simulink model "PubIfDecisionTOS_MDL"  (R2020b)
settings: configuration reference "DspaceConfig" (kept outside this file)
PostLoadFcn:
  | if any(exist('dsrtsu_mdlpostloadfcn', 'file') ~= 0), dsrtsu_mdlpostloadfcn('Execute', bdroot); end
InitFcn:
  | , if any(exist('dsmpb_private', 'file') ~= 0), dsmpb_private('dsmpb_mdlclblib', 'Init', bdroot); end,
undefined symbols (not defined in the file or in its folder): C_TOS_ACCEgoRAxletoFbumplength_m, C_TOS_ACCTargetFront_Flag, C_TOS_AEBJAPedObjDxThre_Val, C_TOS_AEBJAPedObjDyThre_Val, C_TOS_AEBJATargetSize_Val, C_TOS_AEBJAVehObjDxThre_Val, C_TOS_AEBJAVehObjDyThre_Val, C_TOS_AEBJuncPedTargetSize_Val, C_TOS_AEBLatObjDxThre_Val, C_TOS_AEBLatPedDyThre_Val, C_TOS_AEBLatTargetSize_Val, C_TOS_AEBLongTargetInEgoFront_Flag, C_TOS_axAbsGround_Parameter, C_TOS_CameraConfirmedFlag, C_TOS_CNsubjWidth, C_TOS_CurrentLaneCoreMinWidth_Val, C_TOS_CutInProb_Val_Zero, C_TOS_CutOutProb_Val_Zero, C_TOS_D2R_Val, C_TOS_DefaultValueObjectToCenterLine_dy, C_TOS_EgoCarWidth_Val, C_TOS_EgoDxRefPoint_m, C_TOS_EgoRAxletoFbumplength_m, C_TOS_HalfWidthVehicle_Con, C_TOS_HWA_CurrentLaneFlag, C_TOS_HWA_LeftLaneFlag, C_TOS_HWA_MovingDir_Vaild, C_TOS_HWA_MovState_Vaild, C_TOS_HWA_RightLaneFlag, C_TOS_LaneLineCourseErrorFront, C_TOS_LaneLineCourseErrorRear, C_TOS_MotorbikeDefaultWidth_m, C_TOS_NumberOfEffectiveTargets, C_TOS_Obj_Age_Val, C_TOS_Objdx_Constraint_Val, C_TOS_ObjectDefaultWidth_m, C_TOS_ObjInCurrentLane_Val, C_TOS_ObjInCurrentLaneValid, C_TOS_ObjInLeftLaneValid, C_TOS_ObjInRightLaneValid, C_TOS_ObjNotInCurrentLane_Val, C_TOS_ObjNotREElementType, C_TOS_ObjPredictDis_dy_ConstantVal_Zeros, C_TOS_ObjToCenterLine_ConstantVal_Zeros, C_TOS_OFMObjIDInvilad_Val, C_TOS_PIL_LatDisCons_Val_zero, C_TOS_PIL_ObjectCutInFlag_b, C_TOS_PIL_ObjectCutOutFlag_b, C_TOS_PIL_ObjLaneProb_al_Val, C_TOS_PP_ObjFusType_FC_Confirm_b, C_TOS_PP_ObjFusType_FC_FR_Confirm_b, C_TOS_PP_ObjFusType_FR_Confirm_b, C_TOS_RE_80BoolDefault_Val, C_TOS_RE_80Single181Default_Val, C_TOS_RE_80Single255Default_Val, C_TOS_RE_80Uint8Default_Val, C_TOS_RE_D2R, C_TOS_RE_D_180_Val, C_TOS_RE_InvalidObjectID_Val, C_TOS_RE_InvalidTargetChainDir_Val ... (+142)
libraries: simulink x1650, TOS_LIB x361, canfdmsglib x14
(part 61 of 69)

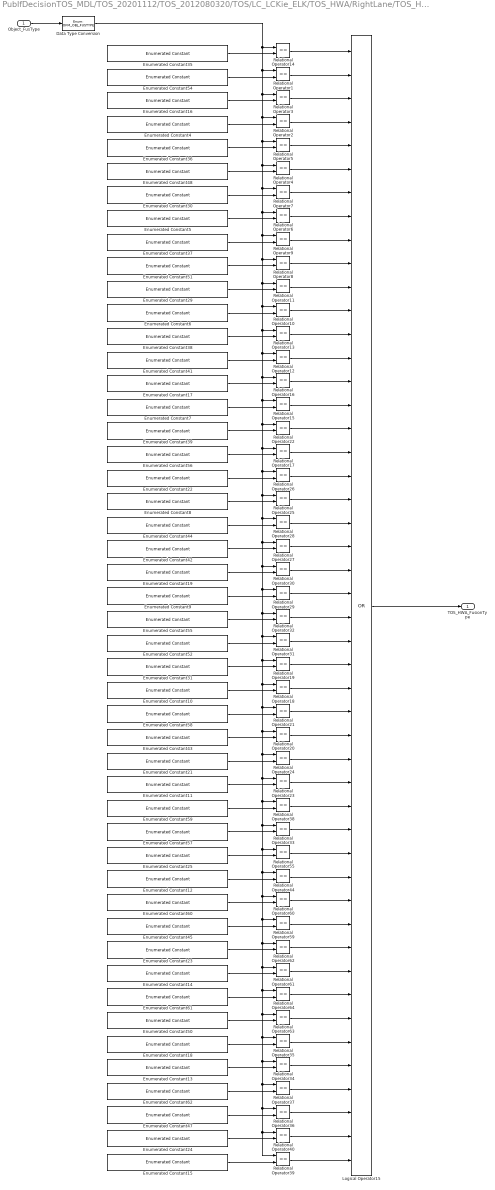
== system PubIfDecisionTOS_MDL/TOS_20201112/TOS_2012080320/TOS/LC_LCKie_ELK/TOS_HWA/RightLane/TOS_HWA_RightLane/TOS_HWA_RightLane/TOS_HWA/HWA_RightLane/HWA_RightLane_Rear/HWA_RightRear_FusionType/FusionType ==
  Object_FusType : Inport
  Data Type Conversion : DataTypeConversion  OutDataTypeStr=Enum: OFM_OBJ_FUSTYPE
  Enumerated Constant10 : simulink/Sources/Enumerated Constant  OutDataTypeStr=Enum: OFM_OBJ_FUSTYPE  Value=OFM_OBJ_FUSTYPE.FC_FR_CR_BR  SampleTime=inf
      settings: AttributesFormatString=OFM_OBJ_FUSTYPE.FC_FR_CR_BR=43
  Enumerated Constant11 : simulink/Sources/Enumerated Constant  OutDataTypeStr=Enum: OFM_OBJ_FUSTYPE  Value=OFM_OBJ_FUSTYPE.FC_FR_CL_CR_BR  SampleTime=inf
      settings: AttributesFormatString=OFM_OBJ_FUSTYPE.FC_FR_CL_CR_BR=47
  Enumerated Constant12 : simulink/Sources/Enumerated Constant  OutDataTypeStr=Enum: OFM_OBJ_FUSTYPE  Value=OFM_OBJ_FUSTYPE.FC_FR_BL_BR  SampleTime=inf
      settings: AttributesFormatString=OFM_OBJ_FUSTYPE.FC_FR_BL_BR=51
  Enumerated Constant13 : simulink/Sources/Enumerated Constant  OutDataTypeStr=Enum: OFM_OBJ_FUSTYPE  Value=OFM_OBJ_FUSTYPE.FC_FR_CR_BL_BR  SampleTime=inf
      settings: AttributesFormatString=OFM_OBJ_FUSTYPE.FC_FR_CR_BL_BR=59
  Enumerated Constant14 : simulink/Sources/Enumerated Constant  OutDataTypeStr=Enum: OFM_OBJ_FUSTYPE  Value=OFM_OBJ_FUSTYPE.FC_FR_CL_BL_BR  SampleTime=inf
      settings: AttributesFormatString=OFM_OBJ_FUSTYPE.FC_FR_CL_BL_BR=55
  Enumerated Constant15 : simulink/Sources/Enumerated Constant  OutDataTypeStr=Enum: OFM_OBJ_FUSTYPE  Value=OFM_OBJ_FUSTYPE.FC_FR_CL_CR_BL_BR  SampleTime=inf
      settings: AttributesFormatString=OFM_OBJ_FUSTYPE.FC_FR_CL_CR_BL_BR=63
  Enumerated Constant16 : simulink/Sources/Enumerated Constant  OutDataTypeStr=Enum: OFM_OBJ_FUSTYPE  Value=OFM_OBJ_FUSTYPE.FR_BL  SampleTime=inf
      settings: AttributesFormatString=OFM_OBJ_FUSTYPE.FR_BL = 18
  Enumerated Constant17 : simulink/Sources/Enumerated Constant  OutDataTypeStr=Enum: OFM_OBJ_FUSTYPE  Value=OFM_OBJ_FUSTYPE.FR_CL_CR_BL  SampleTime=inf
      settings: AttributesFormatString=OFM_OBJ_FUSTYPE.FR_CL_CR_BL = 30
  Enumerated Constant18 : simulink/Sources/Enumerated Constant  OutDataTypeStr=Enum: OFM_OBJ_FUSTYPE  Value=OFM_OBJ_FUSTYPE.FR_CR_BL_BR  SampleTime=inf
      settings: AttributesFormatString=OFM_OBJ_FUSTYPE.FR_CR_BL_BR = 58
  Enumerated Constant19 : simulink/Sources/Enumerated Constant  OutDataTypeStr=Enum: OFM_OBJ_FUSTYPE  Value=OFM_OBJ_FUSTYPE.FR_CL_BR  SampleTime=inf
      settings: AttributesFormatString=OFM_OBJ_FUSTYPE.FR_CL_BR = 38
  Enumerated Constant21 : simulink/Sources/Enumerated Constant  OutDataTypeStr=Enum: OFM_OBJ_FUSTYPE  Value=OFM_OBJ_FUSTYPE.FR_CL_CR_BR  SampleTime=inf
      settings: AttributesFormatString=OFM_OBJ_FUSTYPE.FR_CL_CR_BR = 46
  Enumerated Constant22 : simulink/Sources/Enumerated Constant  OutDataTypeStr=Enum: OFM_OBJ_FUSTYPE  Value=OFM_OBJ_FUSTYPE.FR_BR  SampleTime=inf
      settings: AttributesFormatString=OFM_OBJ_FUSTYPE.FR_BR = 34
  Enumerated Constant23 : simulink/Sources/Enumerated Constant  OutDataTypeStr=Enum: OFM_OBJ_FUSTYPE  Value=OFM_OBJ_FUSTYPE.FR_CL_BL_BR  SampleTime=inf
      settings: AttributesFormatString=OFM_OBJ_FUSTYPE.FR_CL_BL_BR = 54
  Enumerated Constant24 : simulink/Sources/Enumerated Constant  OutDataTypeStr=Enum: OFM_OBJ_FUSTYPE  Value=OFM_OBJ_FUSTYPE.FR_CL_CR_BL_BR  SampleTime=inf
      settings: AttributesFormatString=OFM_OBJ_FUSTYPE.FR_CL_CR_BL_BR = 62
  Enumerated Constant25 : simulink/Sources/Enumerated Constant  OutDataTypeStr=Enum: OFM_OBJ_FUSTYPE  Value=OFM_OBJ_FUSTYPE.FR_BL_BR  SampleTime=inf
      settings: AttributesFormatString=OFM_OBJ_FUSTYPE.FR_BL_BR = 50
  Enumerated Constant29 : simulink/Sources/Enumerated Constant  OutDataTypeStr=Enum: OFM_OBJ_FUSTYPE  Value=OFM_OBJ_FUSTYPE.FR_CR_BL  SampleTime=inf
      settings: AttributesFormatString=OFM_OBJ_FUSTYPE.FR_CR_BL = 26
  Enumerated Constant30 : simulink/Sources/Enumerated Constant  OutDataTypeStr=Enum: OFM_OBJ_FUSTYPE  Value=OFM_OBJ_FUSTYPE.FR_CL_BL  SampleTime=inf
      settings: AttributesFormatString=OFM_OBJ_FUSTYPE.FR_CL_BL = 22
  Enumerated Constant31 : simulink/Sources/Enumerated Constant  OutDataTypeStr=Enum: OFM_OBJ_FUSTYPE  Value=OFM_OBJ_FUSTYPE.FR_CR_BR  SampleTime=inf
      settings: AttributesFormatString=OFM_OBJ_FUSTYPE.FR_CR_BR = 42
  Enumerated Constant35 : simulink/Sources/Enumerated Constant  OutDataTypeStr=Enum: OFM_OBJ_FUSTYPE  Value=OFM_OBJ_FUSTYPE.BL  SampleTime=inf
      settings: AttributesFormatString=OFM_OBJ_FUSTYPE.BL = 16
  Enumerated Constant36 : simulink/Sources/Enumerated Constant  OutDataTypeStr=Enum: OFM_OBJ_FUSTYPE  Value=OFM_OBJ_FUSTYPE.CL_BL  SampleTime=inf
      settings: AttributesFormatString=OFM_OBJ_FUSTYPE.CL_BL=20
  Enumerated Constant37 : simulink/Sources/Enumerated Constant  OutDataTypeStr=Enum: OFM_OBJ_FUSTYPE  Value=OFM_OBJ_FUSTYPE.CR_BL  SampleTime=inf
      settings: AttributesFormatString=OFM_OBJ_FUSTYPE.CR_BL = 24
  Enumerated Constant38 : simulink/Sources/Enumerated Constant  OutDataTypeStr=Enum: OFM_OBJ_FUSTYPE  Value=OFM_OBJ_FUSTYPE.CL_CR_BL  SampleTime=inf
      settings: AttributesFormatString=OFM_OBJ_FUSTYPE.CL_CR_BL=28
  Enumerated Constant39 : simulink/Sources/Enumerated Constant  OutDataTypeStr=Enum: OFM_OBJ_FUSTYPE  Value=OFM_OBJ_FUSTYPE.BR  SampleTime=inf
      settings: AttributesFormatString=OFM_OBJ_FUSTYPE.BR = 32
  Enumerated Constant4 : simulink/Sources/Enumerated Constant  OutDataTypeStr=Enum: OFM_OBJ_FUSTYPE  Value=OFM_OBJ_FUSTYPE.FC_FR_BL  SampleTime=inf
      settings: AttributesFormatString=OFM_OBJ_FUSTYPE.FC_FR_BL=19
  Enumerated Constant41 : simulink/Sources/Enumerated Constant  OutDataTypeStr=Enum: OFM_OBJ_FUSTYPE  Value=OFM_OBJ_FUSTYPE.FC_CL_CR_BL  SampleTime=inf
      settings: AttributesFormatString=OFM_OBJ_FUSTYPE.FC_CL_CR_BL = 29
  Enumerated Constant42 : simulink/Sources/Enumerated Constant  OutDataTypeStr=Enum: OFM_OBJ_FUSTYPE  Value=OFM_OBJ_FUSTYPE.FC_CL_BR  SampleTime=inf
      settings: AttributesFormatString=OFM_OBJ_FUSTYPE.FC_CL_BR = 37
  Enumerated Constant43 : simulink/Sources/Enumerated Constant  OutDataTypeStr=Enum: OFM_OBJ_FUSTYPE  Value=OFM_OBJ_FUSTYPE.FC_CL_CR_BR  SampleTime=inf
      settings: AttributesFormatString=OFM_OBJ_FUSTYPE.FC_CL_CR_BR = 45
  Enumerated Constant44 : simulink/Sources/Enumerated Constant  OutDataTypeStr=Enum: OFM_OBJ_FUSTYPE  Value=OFM_OBJ_FUSTYPE.CL_BR  SampleTime=inf
      settings: AttributesFormatString=OFM_OBJ_FUSTYPE.CL_BR = 36
  Enumerated Constant45 : simulink/Sources/Enumerated Constant  OutDataTypeStr=Enum: OFM_OBJ_FUSTYPE  Value=OFM_OBJ_FUSTYPE.FC_CL_BL_BR  SampleTime=inf
      settings: AttributesFormatString=OFM_OBJ_FUSTYPE.FC_CL_BL_BR = 53
  Enumerated Constant47 : simulink/Sources/Enumerated Constant  OutDataTypeStr=Enum: OFM_OBJ_FUSTYPE  Value=OFM_OBJ_FUSTYPE.FC_CL_CR_BL_BR  SampleTime=inf
      settings: AttributesFormatString=OFM_OBJ_FUSTYPE.FC_CL_CR_BL_BR = 61
  Enumerated Constant48 : simulink/Sources/Enumerated Constant  OutDataTypeStr=Enum: OFM_OBJ_FUSTYPE  Value=OFM_OBJ_FUSTYPE.FC_CL_BL  SampleTime=inf
      settings: AttributesFormatString=OFM_OBJ_FUSTYPE.FC_CL_BL = 21
  Enumerated Constant5 : simulink/Sources/Enumerated Constant  OutDataTypeStr=Enum: OFM_OBJ_FUSTYPE  Value=OFM_OBJ_FUSTYPE.FC_FR_CL_BL  SampleTime=inf
      settings: AttributesFormatString=OFM_OBJ_FUSTYPE.FC_FR_CL_BL=23
  Enumerated Constant50 : simulink/Sources/Enumerated Constant  OutDataTypeStr=Enum: OFM_OBJ_FUSTYPE  Value=OFM_OBJ_FUSTYPE.FC_CR_BL_BR  SampleTime=inf
      settings: AttributesFormatString=OFM_OBJ_FUSTYPE.FC_CR_BL_BR = 57
  Enumerated Constant51 : simulink/Sources/Enumerated Constant  OutDataTypeStr=Enum: OFM_OBJ_FUSTYPE  Value=OFM_OBJ_FUSTYPE.FC_CR_BL  SampleTime=inf
      settings: AttributesFormatString=OFM_OBJ_FUSTYPE.FC_CR_BL = 25
  Enumerated Constant52 : simulink/Sources/Enumerated Constant  OutDataTypeStr=Enum: OFM_OBJ_FUSTYPE  Value=OFM_OBJ_FUSTYPE.FC_CR_BR  SampleTime=inf
      settings: AttributesFormatString=OFM_OBJ_FUSTYPE.FC_CR_BR = 41
  Enumerated Constant54 : simulink/Sources/Enumerated Constant  OutDataTypeStr=Enum: OFM_OBJ_FUSTYPE  Value=OFM_OBJ_FUSTYPE.FC_BL  SampleTime=inf
      settings: AttributesFormatString=OFM_OBJ_FUSTYPE.FC_BL = 17
  Enumerated Constant55 : simulink/Sources/Enumerated Constant  OutDataTypeStr=Enum: OFM_OBJ_FUSTYPE  Value=OFM_OBJ_FUSTYPE.CR_BR  SampleTime=inf
      settings: AttributesFormatString=OFM_OBJ_FUSTYPE.CR_BR = 40
  Enumerated Constant56 : simulink/Sources/Enumerated Constant  OutDataTypeStr=Enum: OFM_OBJ_FUSTYPE  Value=OFM_OBJ_FUSTYPE.FC_BR  SampleTime=inf
      settings: AttributesFormatString=OFM_OBJ_FUSTYPE.FC_BR = 33
  Enumerated Constant57 : simulink/Sources/Enumerated Constant  OutDataTypeStr=Enum: OFM_OBJ_FUSTYPE  Value=OFM_OBJ_FUSTYPE.FC_BL_BR  SampleTime=inf
      settings: AttributesFormatString=OFM_OBJ_FUSTYPE.FC_BL_BR = 49
  Enumerated Constant58 : simulink/Sources/Enumerated Constant  OutDataTypeStr=Enum: OFM_OBJ_FUSTYPE  Value=OFM_OBJ_FUSTYPE.CL_CR_BR  SampleTime=inf
      settings: AttributesFormatString=OFM_OBJ_FUSTYPE.CL_CR_BR = 44
  Enumerated Constant59 : simulink/Sources/Enumerated Constant  OutDataTypeStr=Enum: OFM_OBJ_FUSTYPE  Value=OFM_OBJ_FUSTYPE.BL_BR  SampleTime=inf
      settings: AttributesFormatString=OFM_OBJ_FUSTYPE.BL_BR = 48
  Enumerated Constant6 : simulink/Sources/Enumerated Constant  OutDataTypeStr=Enum: OFM_OBJ_FUSTYPE  Value=OFM_OBJ_FUSTYPE.FC_FR_CR_BL  SampleTime=inf
      settings: AttributesFormatString=OFM_OBJ_FUSTYPE.FC_FR_CR_BL=27
  Enumerated Constant60 : simulink/Sources/Enumerated Constant  OutDataTypeStr=Enum: OFM_OBJ_FUSTYPE  Value=OFM_OBJ_FUSTYPE.CL_BL_BR  SampleTime=inf
      settings: AttributesFormatString=OFM_OBJ_FUSTYPE.CL_BL_BR = 52
  Enumerated Constant61 : simulink/Sources/Enumerated Constant  OutDataTypeStr=Enum: OFM_OBJ_FUSTYPE  Value=OFM_OBJ_FUSTYPE.CR_BL_BR  SampleTime=inf
      settings: AttributesFormatString=OFM_OBJ_FUSTYPE.CR_BL_BR = 56
  Enumerated Constant62 : simulink/Sources/Enumerated Constant  OutDataTypeStr=Enum: OFM_OBJ_FUSTYPE  Value=OFM_OBJ_FUSTYPE.CL_CR_BL_BR  SampleTime=inf
      settings: AttributesFormatString=OFM_OBJ_FUSTYPE.CL_CR_BL_BR = 60
  Enumerated Constant7 : simulink/Sources/Enumerated Constant  OutDataTypeStr=Enum: OFM_OBJ_FUSTYPE  Value=OFM_OBJ_FUSTYPE.FC_FR_CL_CR_BL  SampleTime=inf
      settings: AttributesFormatString=OFM_OBJ_FUSTYPE.FC_FR_CL_CR_BL=31
  Enumerated Constant8 : simulink/Sources/Enumerated Constant  OutDataTypeStr=Enum: OFM_OBJ_FUSTYPE  Value=OFM_OBJ_FUSTYPE.FC_FR_BR  SampleTime=inf
      settings: AttributesFormatString=OFM_OBJ_FUSTYPE.FC_FR_BR=35
  Enumerated Constant9 : simulink/Sources/Enumerated Constant  OutDataTypeStr=Enum: OFM_OBJ_FUSTYPE  Value=OFM_OBJ_FUSTYPE.FC_FR_CL_BR  SampleTime=inf
      settings: AttributesFormatString=OFM_OBJ_FUSTYPE.FC_FR_CL_BR=39
  Logical Operator15 : Logic  Operator=OR  Inputs=48  AllPortsSameDT=off  OutDataTypeStr=boolean
  Relational Operator{1..40,44,55,59..64} (48 alike) : RelationalOperator  Operator===  OutDataTypeStr=boolean  RndMeth=Nearest
  TOS_HWA_FusionType : Outport
  wires:
  Relational Operator29/1 -> Logical Operator15/24
  Enumerated Constant50/1 -> Relational Operator63/2
  Enumerated Constant15/1 -> Relational Operator39/2
  Relational Operator8/1 -> Logical Operator15/10
  Relational Operator27/1 -> Logical Operator15/22
  Relational Operator7/1 -> Logical Operator15/7
  Enumerated Constant54/1 -> Relational Operator1/2
  Enumerated Constant58/1 -> Relational Operator21/2
  Relational Operator16/1 -> Logical Operator15/15
  Enumerated Constant44/1 -> Relational Operator28/2
  Enumerated Constant48/1 -> Relational Operator4/2
  Enumerated Constant23/1 -> Relational Operator62/2
  Relational Operator28/1 -> Logical Operator15/21
  Logical Operator15/1 -> TOS_HWA_FusionType/1
  Relational Operator23/1 -> Logical Operator15/32
  Relational Operator13/1 -> Logical Operator15/13
  Relational Operator3/1 -> Logical Operator15/3
  Relational Operator38/1 -> Logical Operator15/33
  Enumerated Constant16/1 -> Relational Operator3/2
  Enumerated Constant4/1 -> Relational Operator2/2
  Relational Operator9/1 -> Logical Operator15/9
  Enumerated Constant57/1 -> Relational Operator33/2
  Relational Operator33/1 -> Logical Operator15/34
  Enumerated Constant19/1 -> Relational Operator30/2
  Enumerated Constant30/1 -> Relational Operator7/2
  Relational Operator17/1 -> Logical Operator15/18
  Relational Operator25/1 -> Logical Operator15/20
  Relational Operator1/1 -> Logical Operator15/2
  Enumerated Constant41/1 -> Relational Operator12/2
  Enumerated Constant7/1 -> Relational Operator15/2
  Relational Operator64/1 -> Logical Operator15/41
  Relational Operator35/1 -> Logical Operator15/43
  Relational Operator63/1 -> Logical Operator15/42
  Enumerated Constant6/1 -> Relational Operator10/2
  Relational Operator44/1 -> Logical Operator15/36
  Relational Operator34/1 -> Logical Operator15/44
  Relational Operator15/1 -> Logical Operator15/16
  Relational Operator59/1 -> Logical Operator15/38
  Enumerated Constant22/1 -> Relational Operator26/2
  Relational Operator22/1 -> Logical Operator15/17
  Enumerated Constant35/1 -> Relational Operator14/2
  Enumerated Constant37/1 -> Relational Operator9/2
  Enumerated Constant59/1 -> Relational Operator38/2
  Enumerated Constant21/1 -> Relational Operator24/2
  Relational Operator6/1 -> Logical Operator15/8
  Enumerated Constant9/1 -> Relational Operator29/2
  Relational Operator11/1 -> Logical Operator15/11
  Relational Operator26/1 -> Logical Operator15/19
  Relational Operator60/1 -> Logical Operator15/37
  Enumerated Constant45/1 -> Relational Operator59/2
  Relational Operator18/1 -> Logical Operator15/28
  Enumerated Constant12/1 -> Relational Operator44/2
  Enumerated Constant11/1 -> Relational Operator23/2
  Enumerated Constant14/1 -> Relational Operator61/2
  Relational Operator36/1 -> Logical Operator15/46
  Relational Operator20/1 -> Logical Operator15/30
  Enumerated Constant31/1 -> Relational Operator19/2
  Enumerated Constant55/1 -> Relational Operator32/2
  Enumerated Constant43/1 -> Relational Operator20/2
  Relational Operator61/1 -> Logical Operator15/40
  Relational Operator19/1 -> Logical Operator15/27
  Enumerated Constant18/1 -> Relational Operator35/2
  Enumerated Constant5/1 -> Relational Operator6/2
  Relational Operator10/1 -> Logical Operator15/12
  Enumerated Constant25/1 -> Relational Operator55/2
  Relational Operator24/1 -> Logical Operator15/31
  Relational Operator21/1 -> Logical Operator15/29
  Enumerated Constant60/1 -> Relational Operator60/2
  Enumerated Constant61/1 -> Relational Operator64/2
  Relational Operator40/1 -> Logical Operator15/47
  Relational Operator2/1 -> Logical Operator15/4
  Relational Operator4/1 -> Logical Operator15/6
  Enumerated Constant8/1 -> Relational Operator25/2
  Enumerated Constant47/1 -> Relational Operator36/2
  Enumerated Constant13/1 -> Relational Operator34/2
  Enumerated Constant38/1 -> Relational Operator13/2
  Relational Operator37/1 -> Logical Operator15/45
  Object_FusType/1 -> Data Type Conversion/1
  Relational Operator5/1 -> Logical Operator15/5
  Relational Operator32/1 -> Logical Operator15/25
  Relational Operator39/1 -> Logical Operator15/48
  Enumerated Constant24/1 -> Relational Operator40/2
  Enumerated Constant51/1 -> Relational Operator8/2
  Enumerated Constant29/1 -> Relational Operator11/2
  Enumerated Constant56/1 -> Relational Operator17/2
  Enumerated Constant52/1 -> Relational Operator31/2
  Enumerated Constant10/1 -> Relational Operator18/2
  Relational Operator30/1 -> Logical Operator15/23
  Enumerated Constant17/1 -> Relational Operator16/2
  Relational Operator62/1 -> Logical Operator15/39
  Enumerated Constant42/1 -> Relational Operator27/2
  Enumerated Constant62/1 -> Relational Operator37/2
  Relational Operator31/1 -> Logical Operator15/26
  Relational Operator55/1 -> Logical Operator15/35
  Enumerated Constant36/1 -> Relational Operator5/2
  Relational Operator14/1 -> Logical Operator15/1
  Enumerated Constant39/1 -> Relational Operator22/2
  Data Type Conversion/1 -> Relational Operator1/1, Relational Operator3/1, Relational Operator2/1, Relational Operator5/1, Relational Operator4/1, Relational Operator7/1, Relational Operator6/1, Relational Operator9/1, Relational Operator8/1, Relational Operator11/1, Relational Operator10/1, Relational Operator13/1, Relational Operator12/1, Relational Operator16/1, Relational Operator15/1, Relational Operator22/1, Relational Operator17/1, Relational Operator26/1, Relational Operator25/1, Relational Operator28/1, Relational Operator27/1, Relational Operator30/1, Relational Operator29/1, Relational Operator32/1, Relational Operator31/1, Relational Operator19/1, Relational Operator18/1, Relational Operator21/1, Relational Operator20/1, Relational Operator24/1, Relational Operator23/1, Relational Operator38/1, Relational Operator33/1, Relational Operator55/1, Relational Operator44/1, Relational Operator60/1, Relational Operator59/1, Relational Operator62/1, Relational Operator61/1, Relational Operator64/1, Relational Operator63/1, Relational Operator34/1, Relational Operator37/1, Relational Operator36/1, Relational Operator40/1, Relational Operator39/1, Relational Operator35/1, Relational Operator14/1
  Relational Operator12/1 -> Logical Operator15/14

== system PubIfDecisionTOS_MDL/TOS_20201112/TOS_2012080320/TOS/AEB/TOS_AEBLong/AEBLong_Confirm/AEBLong/AEBLong_TrgConfirm/AEBLongTrgJudg/TOS_AEBLong_TargetMovingDir/ObjMovingDirSignalProcessing1/MappingObjInCurveLaneVXVY/ObjectInCurveLaneMappingVXVY/BaseObjDx_C1_C2_Calculate ==
  Object_DX : Inport
  line01_C1 : Inport  Port=2
  line01_C2 : Inport  Port=3
  line01_dDisStart : Inport  Port=4
  line01_dDisEnd : Inport  Port=5
  line02_C1 : Inport  Port=6
  line02_C2 : Inport  Port=7
  line02_dDisStart : Inport  Port=8
  line02_dDisEnd : Inport  Port=9
  line03_C1 : Inport  Port=10
  line03_C2 : Inport  Port=11
  line03_dDisStart : Inport  Port=12
  line03_dDisEnd : Inport  Port=13
  line04_C1 : Inport  Port=14
  line04_C2 : Inport  Port=15
  line04_dDisStart : Inport  Port=16
  line04_dDisEnd : Inport  Port=17
  line05_C1 : Inport  Port=18
  line05_C2 : Inport  Port=19
  line05_dDisStart : Inport  Port=20
  line05_dDisEnd : Inport  Port=21
  line06_C1 : Inport  Port=22
  line06_C2 : Inport  Port=23
  line06_dDisStart : Inport  Port=24
  line06_dDisEnd : Inport  Port=25
  Bus Creator{,1..6} (7 alike) : BusCreator  Inputs=2
  Constant1 : Constant  Value=P_TOS_MovingDirJudge_C1Default_Val  OutDataTypeStr=single
      settings: AttributesFormatString=P_TOS_MovingDirJudge_C1Default_Val = 0
  Constant2 : Constant  Value=P_TOS_MovingDirJudge_C2Default_Val  OutDataTypeStr=single
      settings: AttributesFormatString=P_TOS_MovingDirJudge_C2Default_Val = 0
  Switch{,1..5} (6 alike) : Switch  Criteria=u2 ~= 0  OutDataTypeStr=single
  line01_DisJudge : Subsystem
  line02_DisJudge : Subsystem
  line03_DisJudge : Subsystem
  line04_DisJudge : Subsystem
  line05_DisJudge : Subsystem
  line06_DisJudge : Subsystem
  BaseObjDx_C1_C2 : Outport  OutDataTypeStr=single
  wires:
  line05_dDisEnd/1 -> line05_DisJudge/3(line05_dDisEnd)
  line04_dDisStart/1 -> line04_DisJudge/2(line04_dDisStart)
  line06_DisJudge/1(line06_DisJudge) -> Switch5/2
  line06_dDisStart/1 -> line06_DisJudge/2(line06_dDisStart)
  [Object_DX] -> line06_DisJudge/1(Object_DX)
  line03_DisJudge/1(line03_DisJudge) -> Switch2/2
  line03_dDisStart/1 -> line03_DisJudge/2(line03_dDisStart)
  line02_DisJudge/1(line02_DisJudge) -> Switch1/2
  Bus Creator6/1 -> Switch5/3
  Bus Creator5/1 -> Switch5/1
  [Object_DX] -> line03_DisJudge/1(Object_DX)
  line03_dDisEnd/1 -> line03_DisJudge/3(line03_dDisEnd)
  [Object_DX] -> line02_DisJudge/1(Object_DX)
  line05_DisJudge/1(line05_DisJudge) -> Switch4/2
  line04_DisJudge/1(line04_DisJudge) -> Switch3/2
  line02_dDisEnd/1 -> line02_DisJudge/3(line02_dDisEnd)
  line06_dDisEnd/1 -> line06_DisJudge/3(line06_dDisEnd)
  line04_dDisEnd/1 -> line04_DisJudge/3(line04_dDisEnd)
  line02_dDisStart/1 -> line02_DisJudge/2(line02_dDisStart)
  [Object_DX] -> line05_DisJudge/1(Object_DX)
  line05_dDisStart/1 -> line05_DisJudge/2(line05_dDisStart)
  [Object_DX] -> line04_DisJudge/1(Object_DX)
  Switch5/1 -> Switch4/3
  Bus Creator1/1 -> Switch1/1
  Object_DX/1 -> [Object_DX], line01_DisJudge/1(Object_DX)
  Bus Creator2/1 -> Switch2/1
  line01_DisJudge/1(line01_DisJudge) -> Switch/2
  Switch4/1 -> Switch3/3
  Switch3/1 -> Switch2/3
  Switch1/1 -> Switch/3
  line01_dDisStart/1 -> line01_DisJudge/2(line01_dDisStart)
  Bus Creator4/1 -> Switch4/1
  Switch2/1 -> Switch1/3
  Switch/1 -> BaseObjDx_C1_C2/1
  Bus Creator3/1 -> Switch3/1
  line01_dDisEnd/1 -> line01_DisJudge/3(line01_dDisEnd)
  Bus Creator/1 -> Switch/1
  line01_C2/1 -> Bus Creator/2  "C2"
  line01_C1/1 -> Bus Creator/1  "C1"
  line02_C2/1 -> Bus Creator1/2  "C2"
  line02_C1/1 -> Bus Creator1/1  "C1"
  line03_C2/1 -> Bus Creator2/2  "C2"
  line03_C1/1 -> Bus Creator2/1  "C1"
  line04_C2/1 -> Bus Creator3/2  "C2"
  line04_C1/1 -> Bus Creator3/1  "C1"
  line05_C2/1 -> Bus Creator4/2  "C2"
  line05_C1/1 -> Bus Creator4/1  "C1"
  line06_C2/1 -> Bus Creator5/2  "C2"
  line06_C1/1 -> Bus Creator5/1  "C1"
  Constant2/1 -> Bus Creator6/2  "C2"
  Constant1/1 -> Bus Creator6/1  "C1"

== system PubIfDecisionTOS_MDL/TOS_20201112/TOS_2012080320/TOS/AEB/TOS_AEBLong/AEBLong_Confirm/AEBLong/AEBLong_TrgConfirm/AEBLongTrgJudg/TOS_AEBLong_TargetMovingDir/ObjMovingDirSignalProcessing1/MappingObjInCurveLaneVXVY/ObjectInCurveLaneMappingVXVY/Object_MappingVXVYCalculate ==
  note: 直道，VXVY不做处理
  note: 判断目标所在的那段车道线是否为直道
  note: 弯道，VXVY做映射处理
  Object_VX : Inport
  Object_VY : Inport  Port=2
  BaseObjDx_C1_C2 : Inport  Port=3  OutDataTypeStr=single
  Bus Creator : BusCreator  Inputs=3
  Bus Selector1 : BusSelector  OutputSignals=BaseObjDx_C1_C2.C2
  Bus Selector2 : BusSelector  OutputSignals=Object_VX,Object_VY,BaseObjDx_C1_C2.C1
  Bus Selector3 : BusSelector  OutputSignals=Object_VX,Object_VY
  If : If  IfExpression=u1 <= P_TOS_CurveLaneC2Thre_Val
  If Action Subsystem : Subsystem  TreatAsAtomicUnit=on
  If Action Subsystem1 : Subsystem  TreatAsAtomicUnit=on
  Merge : Merge
  Merge1 : Merge
  Object_MappingVX : Outport
  Object_MappingVY : Outport  Port=2
  wires:
  Merge/1 -> Object_MappingVX/1
  Bus Creator/1 -> Bus Selector1/1, Bus Selector3/1, Bus Selector2/1
  Bus Selector1/1 -> If/1  "<C2>"
  If/1 -> If Action Subsystem/Action
  If Action Subsystem/1(StraightLaneMappingVX) -> Merge/2
  If/2 -> If Action Subsystem1/Action
  Object_VX/1 -> Bus Creator/1  "Object_VX"
  Object_VY/1 -> Bus Creator/2  "Object_VY"
  BaseObjDx_C1_C2/1 -> Bus Creator/3  "BaseObjDx_C1_C2"
  Bus Selector2/1 -> If Action Subsystem1/1(Object_VX)  "<Object_VX>"
  Bus Selector2/2 -> If Action Subsystem1/2(Object_VY)  "<Object_VY>"
  Bus Selector2/3 -> If Action Subsystem1/3(BaseObjDx_C1)  "<C1>"
  If Action Subsystem1/1(CurveLaneMappingVX) -> [CurveLaneMappingVX]
  If Action Subsystem1/2(CurveLaneMappingVY) -> [CurveLaneMappingVY]
  [CurveLaneMappingVX] -> Merge/1
  [CurveLaneMappingVY] -> Merge1/1
  If Action Subsystem/2(StraightLaneMappingVY) -> Merge1/2
  Merge1/1 -> Object_MappingVY/1
  Bus Selector3/1 -> If Action Subsystem/1(Object_VX)  "<Object_VX>"
  Bus Selector3/2 -> If Action Subsystem/2(Object_VY)  "<Object_VY>"

== system PubIfDecisionTOS_MDL/TOS_20201112/TOS_2012080320/TOS/AEB/TOS_AEBLong/AEBLong_Confirm/AEBLong/AEBLong_TrgConfirm/AEBLongTrgJudg/TOS_AEBLong_TargetMovingDir/ObjMovingDirSignalProcessing1/MappingObjInCurveLaneVXVY/ObjectVYVXAngle/Object_VXMeanFilt ==
  Object_VX : Inport
  Add : Sum  Inputs=+++++
  Constant : Constant  Value=5
  Delay : Delay
  Delay1 : Delay  DelayLength=1
  Delay2 : Delay  DelayLength=3
  Delay3 : Delay  DelayLength=4
  Divide : Product  Inputs=*/
  ObjectVXFilt : Outport
  wires:
  Divide/1 -> ObjectVXFilt/1
  Constant/1 -> Divide/2
  Add/1 -> Divide/1
  Delay/1 -> Add/3
  Delay2/1 -> Add/4
  Delay3/1 -> Add/5
  Object_VX/1 -> Delay3/1, Delay2/1, Delay/1, Delay1/1, Add/1
  Delay1/1 -> Add/2

== system PubIfDecisionTOS_MDL/TOS_20201112/TOS_2012080320/TOS/AEB/TOS_AEBLong/AEBLong_Confirm/AEBLong/AEBLong_TrgConfirm/AEBLongTrgJudg/TOS_AEBLong_TargetMovingDir/ObjMovingDirSignalProcessing1/MappingObjInCurveLaneVXVY/ObjectVYVXAngle/Object_VYMeanFilt ==
  Object_VY : Inport
  Add : Sum  Inputs=+++++
  Constant : Constant  Value=5
  Delay : Delay
  Delay1 : Delay  DelayLength=1
  Delay2 : Delay  DelayLength=3
  Delay3 : Delay  DelayLength=4
  Divide : Product  Inputs=*/
  ObjectVYFilt : Outport
  wires:
  Delay1/1 -> Add/2
  Object_VY/1 -> Add/1, Delay1/1, Delay/1, Delay2/1, Delay3/1
  Delay3/1 -> Add/5
  Delay2/1 -> Add/4
  Delay/1 -> Add/3
  Add/1 -> Divide/1
  Constant/1 -> Divide/2
  Divide/1 -> ObjectVYFilt/1

== system PubIfDecisionTOS_MDL/TOS_20201112/TOS_2012080320/TOS/AEB/TOS_AEBLong/AEBLong_Confirm/AEBLong/AEBLong_TrgConfirm/AEBLongTrgJudg/TOS_AEBLong_TargetMovingDir/ObjMovingDirSignalProcessing1/MappingObjInCurveLaneVXVY/ObjectVYVXAngle/Object_VYVXAngle ==
  ObjectVYFilt : Inport
  ObjectVXFilt : Inport  Port=2
  Constant : Constant  Value=C_TOS_D2R_Val
      settings: AttributesFormatString=C_TOS_D2R_Val = 360
  If : If  NumInputs=2  IfExpression=(u1 >= 0) & (u2 >= 0)  ElseIfExpressions=(u1 >= 0) & (u2 < 0),(u1 < 0) & (u2 >= 0)
  If Action Subsystem : Subsystem  TreatAsAtomicUnit=on
  If Action Subsystem1 : Subsystem  TreatAsAtomicUnit=on
  If Action Subsystem2 : Subsystem  TreatAsAtomicUnit=on
  If Action Subsystem3 : Subsystem  TreatAsAtomicUnit=on
  Merge : Merge  Inputs=4
  Product : Product
  VYVXAngle0 : Subsystem
  Object_VYVXAngle : Outport
  wires:
  ObjectVXFilt/1 -> If/2, VYVXAngle0/2(ObjectVXFilt)
  Merge/1 -> Product/1
  ObjectVYFilt/1 -> If/1, VYVXAngle0/1(ObjectVYFilt)
  If Action Subsystem/1(Object_VYVXAngle) -> Merge/1
  If/1 -> If Action Subsystem/Action
  If/2 -> If Action Subsystem1/Action
  If Action Subsystem1/1(Object_VYVXAngle) -> Merge/2
  If Action Subsystem2/1(Object_VYVXAngle) -> Merge/3
  If Action Subsystem3/1(Object_VYVXAngle) -> Merge/4
  If/3 -> If Action Subsystem2/Action
  If/4 -> If Action Subsystem3/Action
  VYVXAngle0/1(Object_VYVXAngle0) -> If Action Subsystem3/1(Object_VYVXAngle0), If Action Subsystem2/1(Object_VYVXAngle0), If Action Subsystem1/1(Object_VYVXAngle0), If Action Subsystem/1(Object_VYVXAngle0)
  Product/1 -> Object_VYVXAngle/1
  Constant/1 -> Product/2

== system PubIfDecisionTOS_MDL/TOS_20201112/TOS_2012080320/TOS/AEB/TOS_AEBLong/AEBLong_Confirm/AEBLong/AEBLong_TrgConfirm/AEBLongTrgJudg/TOS_AEBLong_TargetMovingDir/ObjMovingDirSignalProcessing1/MappingObjInCurveLaneVXVY/ObjectInCurveLaneMappingVXVY/BaseObjDx_C1_C2_Calculate/line01_DisJudge ==
  Object_DX : Inport
  line01_dDisStart : Inport  Port=2
  line01_dDisEnd : Inport  Port=3
  Logical Operator : Logic  AllPortsSameDT=off  OutDataTypeStr=boolean
  Relational Operator : RelationalOperator  OutDataTypeStr=boolean  RndMeth=Nearest
  Relational Operator1 : RelationalOperator  Operator=<  OutDataTypeStr=boolean  RndMeth=Nearest
  line01_DisJudge : Outport
  wires:
  Logical Operator/1 -> line01_DisJudge/1
  Relational Operator1/1 -> Logical Operator/2
  Relational Operator/1 -> Logical Operator/1
  Object_DX/1 -> Relational Operator/1, Relational Operator1/1
  line01_dDisStart/1 -> Relational Operator/2
  line01_dDisEnd/1 -> Relational Operator1/2

== system PubIfDecisionTOS_MDL/TOS_20201112/TOS_2012080320/TOS/AEB/TOS_AEBLong/AEBLong_Confirm/AEBLong/AEBLong_TrgConfirm/AEBLongTrgJudg/TOS_AEBLong_TargetMovingDir/ObjMovingDirSignalProcessing1/MappingObjInCurveLaneVXVY/ObjectInCurveLaneMappingVXVY/BaseObjDx_C1_C2_Calculate/line02_DisJudge ==
  Object_DX : Inport
  line02_dDisStart : Inport  Port=2
  line02_dDisEnd : Inport  Port=3
  Logical Operator : Logic  AllPortsSameDT=off  OutDataTypeStr=boolean
  Relational Operator : RelationalOperator  OutDataTypeStr=boolean  RndMeth=Nearest
  Relational Operator1 : RelationalOperator  Operator=<  OutDataTypeStr=boolean  RndMeth=Nearest
  line02_DisJudge : Outport
  wires:
  line02_dDisEnd/1 -> Relational Operator1/2
  line02_dDisStart/1 -> Relational Operator/2
  Object_DX/1 -> Relational Operator1/1, Relational Operator/1
  Relational Operator/1 -> Logical Operator/1
  Relational Operator1/1 -> Logical Operator/2
  Logical Operator/1 -> line02_DisJudge/1

== system PubIfDecisionTOS_MDL/TOS_20201112/TOS_2012080320/TOS/AEB/TOS_AEBLong/AEBLong_Confirm/AEBLong/AEBLong_TrgConfirm/AEBLongTrgJudg/TOS_AEBLong_TargetMovingDir/ObjMovingDirSignalProcessing1/MappingObjInCurveLaneVXVY/ObjectInCurveLaneMappingVXVY/BaseObjDx_C1_C2_Calculate/line03_DisJudge ==
  Object_DX : Inport
  line03_dDisStart : Inport  Port=2
  line03_dDisEnd : Inport  Port=3
  Logical Operator : Logic  AllPortsSameDT=off  OutDataTypeStr=boolean
  Relational Operator : RelationalOperator  OutDataTypeStr=boolean  RndMeth=Nearest
  Relational Operator1 : RelationalOperator  Operator=<  OutDataTypeStr=boolean  RndMeth=Nearest
  line03_DisJudge : Outport
  wires:
  Logical Operator/1 -> line03_DisJudge/1
  Relational Operator1/1 -> Logical Operator/2
  Relational Operator/1 -> Logical Operator/1
  Object_DX/1 -> Relational Operator/1, Relational Operator1/1
  line03_dDisStart/1 -> Relational Operator/2
  line03_dDisEnd/1 -> Relational Operator1/2

== system PubIfDecisionTOS_MDL/TOS_20201112/TOS_2012080320/TOS/AEB/TOS_AEBLong/AEBLong_Confirm/AEBLong/AEBLong_TrgConfirm/AEBLongTrgJudg/TOS_AEBLong_TargetMovingDir/ObjMovingDirSignalProcessing1/MappingObjInCurveLaneVXVY/ObjectInCurveLaneMappingVXVY/BaseObjDx_C1_C2_Calculate/line04_DisJudge ==
  Object_DX : Inport
  line04_dDisStart : Inport  Port=2
  line04_dDisEnd : Inport  Port=3
  Logical Operator : Logic  AllPortsSameDT=off  OutDataTypeStr=boolean
  Relational Operator : RelationalOperator  OutDataTypeStr=boolean  RndMeth=Nearest
  Relational Operator1 : RelationalOperator  Operator=<  OutDataTypeStr=boolean  RndMeth=Nearest
  line04_DisJudge : Outport
  wires:
  line04_dDisEnd/1 -> Relational Operator1/2
  line04_dDisStart/1 -> Relational Operator/2
  Object_DX/1 -> Relational Operator1/1, Relational Operator/1
  Relational Operator/1 -> Logical Operator/1
  Relational Operator1/1 -> Logical Operator/2
  Logical Operator/1 -> line04_DisJudge/1

== system PubIfDecisionTOS_MDL/TOS_20201112/TOS_2012080320/TOS/AEB/TOS_AEBLong/AEBLong_Confirm/AEBLong/AEBLong_TrgConfirm/AEBLongTrgJudg/TOS_AEBLong_TargetMovingDir/ObjMovingDirSignalProcessing1/MappingObjInCurveLaneVXVY/ObjectInCurveLaneMappingVXVY/BaseObjDx_C1_C2_Calculate/line05_DisJudge ==
  Object_DX : Inport
  line05_dDisStart : Inport  Port=2
  line05_dDisEnd : Inport  Port=3
  Logical Operator : Logic  AllPortsSameDT=off  OutDataTypeStr=boolean
  Relational Operator : RelationalOperator  OutDataTypeStr=boolean  RndMeth=Nearest
  Relational Operator1 : RelationalOperator  Operator=<  OutDataTypeStr=boolean  RndMeth=Nearest
  line05_DisJudge : Outport
  wires:
  Logical Operator/1 -> line05_DisJudge/1
  Relational Operator1/1 -> Logical Operator/2
  Relational Operator/1 -> Logical Operator/1
  Object_DX/1 -> Relational Operator/1, Relational Operator1/1
  line05_dDisStart/1 -> Relational Operator/2
  line05_dDisEnd/1 -> Relational Operator1/2

== system PubIfDecisionTOS_MDL/TOS_20201112/TOS_2012080320/TOS/AEB/TOS_AEBLong/AEBLong_Confirm/AEBLong/AEBLong_TrgConfirm/AEBLongTrgJudg/TOS_AEBLong_TargetMovingDir/ObjMovingDirSignalProcessing1/MappingObjInCurveLaneVXVY/ObjectInCurveLaneMappingVXVY/BaseObjDx_C1_C2_Calculate/line06_DisJudge ==
  Object_DX : Inport
  line06_dDisStart : Inport  Port=2
  line06_dDisEnd : Inport  Port=3
  Logical Operator : Logic  AllPortsSameDT=off  OutDataTypeStr=boolean
  Relational Operator : RelationalOperator  OutDataTypeStr=boolean  RndMeth=Nearest
  Relational Operator1 : RelationalOperator  Operator=<  OutDataTypeStr=boolean  RndMeth=Nearest
  line06_DisJudge : Outport
  wires:
  line06_dDisEnd/1 -> Relational Operator1/2
  line06_dDisStart/1 -> Relational Operator/2
  Object_DX/1 -> Relational Operator1/1, Relational Operator/1
  Relational Operator/1 -> Logical Operator/1
  Relational Operator1/1 -> Logical Operator/2
  Logical Operator/1 -> line06_DisJudge/1

== system PubIfDecisionTOS_MDL/TOS_20201112/TOS_2012080320/TOS/AEB/TOS_AEBLong/AEBLong_Confirm/AEBLong/AEBLong_TrgConfirm/AEBLongTrgJudg/TOS_AEBLong_TargetMovingDir/ObjMovingDirSignalProcessing1/MappingObjInCurveLaneVXVY/ObjectInCurveLaneMappingVXVY/Object_MappingVXVYCalculate/If Action Subsystem ==
  Object_VX : Inport
  Object_VY : Inport  Port=2
  Action Port : ActionPort
  StraightLaneMappingVX : Outport
  StraightLaneMappingVY : Outport  Port=2
  wires:
  Object_VY/1 -> StraightLaneMappingVY/1
  Object_VX/1 -> StraightLaneMappingVX/1

== system PubIfDecisionTOS_MDL/TOS_20201112/TOS_2012080320/TOS/AEB/TOS_AEBLong/AEBLong_Confirm/AEBLong/AEBLong_TrgConfirm/AEBLongTrgJudg/TOS_AEBLong_TargetMovingDir/ObjMovingDirSignalProcessing1/MappingObjInCurveLaneVXVY/ObjectInCurveLaneMappingVXVY/Object_MappingVXVYCalculate/If Action Subsystem1 ==
  Object_VX : Inport
  Object_VY : Inport  Port=2
  BaseObjDx_C1 : Inport  Port=3
  Action Port : ActionPort
  Bus Selector : BusSelector  OutputSignals=C1
  MappingVX_VY : Subsystem
  cosC1Calculate_Taylor : Subsystem
  sinC1Calculate_Taylor : Subsystem
  CurveLaneMappingVX : Outport
  CurveLaneMappingVY : Outport  Port=2
  wires:
  MappingVX_VY/1(MappingVX) -> CurveLaneMappingVX/1
  BaseObjDx_C1/1 -> Bus Selector/1
  Object_VX/1 -> MappingVX_VY/1(Object_VX)
  Object_VY/1 -> MappingVX_VY/2(Object_VY)
  cosC1Calculate_Taylor/1(cosC1) -> MappingVX_VY/4(cosc1)
  sinC1Calculate_Taylor/1(sinC1) -> MappingVX_VY/3(sinc1)
  Bus Selector/1 -> sinC1Calculate_Taylor/1(C1_BaseObjDx), cosC1Calculate_Taylor/1(C1_BaseObjDx)  "<C1>"
  MappingVX_VY/2(MappingVY) -> CurveLaneMappingVY/1

== system PubIfDecisionTOS_MDL/TOS_20201112/TOS_2012080320/TOS/AEB/TOS_AEBLong/AEBLong_Confirm/AEBLong/AEBLong_TrgConfirm/AEBLongTrgJudg/TOS_AEBLong_TargetMovingDir/ObjMovingDirSignalProcessing1/MappingObjInCurveLaneVXVY/ObjectVYVXAngle/Object_VYVXAngle/If Action Subsystem ==
  Object_VYVXAngle0 : Inport
  Action Port : ActionPort
  Object_VYVXAngle : Outport
  wires:
  Object_VYVXAngle0/1 -> Object_VYVXAngle/1

== system PubIfDecisionTOS_MDL/TOS_20201112/TOS_2012080320/TOS/AEB/TOS_AEBLong/AEBLong_Confirm/AEBLong/AEBLong_TrgConfirm/AEBLongTrgJudg/TOS_AEBLong_TargetMovingDir/ObjMovingDirSignalProcessing1/MappingObjInCurveLaneVXVY/ObjectVYVXAngle/Object_VYVXAngle/If Action Subsystem1 ==
  note: VY>0,VX<0时，Angle0<0
      | Angle=3.14 + Angle0
  Object_VYVXAngle0 : Inport
  Action Port : ActionPort
  Add : Sum
  Constant : Constant  Value=P_TOS_VYVXAngleMax_Val
      settings: AttributesFormatString=P_TOS_VYVXAngleMax_Val = 3.14
  Object_VYVXAngle : Outport
  wires:
  Constant/1 -> Add/2
  Object_VYVXAngle0/1 -> Add/1
  Add/1 -> Object_VYVXAngle/1

== system PubIfDecisionTOS_MDL/TOS_20201112/TOS_2012080320/TOS/AEB/TOS_AEBLong/AEBLong_Confirm/AEBLong/AEBLong_TrgConfirm/AEBLongTrgJudg/TOS_AEBLong_TargetMovingDir/ObjMovingDirSignalProcessing1/MappingObjInCurveLaneVXVY/ObjectVYVXAngle/Object_VYVXAngle/If Action Subsystem2 ==
  Object_VYVXAngle0 : Inport
  Action Port : ActionPort
  Object_VYVXAngle : Outport
  wires:
  Object_VYVXAngle0/1 -> Object_VYVXAngle/1

== system PubIfDecisionTOS_MDL/TOS_20201112/TOS_2012080320/TOS/AEB/TOS_AEBLong/AEBLong_Confirm/AEBLong/AEBLong_TrgConfirm/AEBLongTrgJudg/TOS_AEBLong_TargetMovingDir/ObjMovingDirSignalProcessing1/MappingObjInCurveLaneVXVY/ObjectVYVXAngle/Object_VYVXAngle/If Action Subsystem3 ==
  note: VY<0,VX<0时，Angle0>0
      | Angle=-3.14 + Angle0
  Object_VYVXAngle0 : Inport
  Action Port : ActionPort
  Add : Sum
  Constant : Constant  Value=P_TOS_VYVXAngleMin_Val
      settings: AttributesFormatString=P_TOS_VYVXAngleMax_Val = -3.14
  Object_VYVXAngle : Outport
  wires:
  Constant/1 -> Add/2
  Object_VYVXAngle0/1 -> Add/1
  Add/1 -> Object_VYVXAngle/1

== system PubIfDecisionTOS_MDL/TOS_20201112/TOS_2012080320/TOS/AEB/TOS_AEBLong/AEBLong_Confirm/AEBLong/AEBLong_TrgConfirm/AEBLongTrgJudg/TOS_AEBLong_TargetMovingDir/ObjMovingDirSignalProcessing1/MappingObjInCurveLaneVXVY/ObjectVYVXAngle/Object_VYVXAngle/VYVXAngle0 ==
  ObjectVYFilt : Inport
  ObjectVXFilt : Inport  Port=2
  Divide : Product  Inputs=*/
  Fcn : Fcn  Expr=atan(u)
  Saturation : Saturate  UpperLimit=300  LowerLimit=0.001
  Object_VYVXAngle0 : Outport
  wires:
  Divide/1 -> Fcn/1
  Saturation/1 -> Divide/2
  ObjectVXFilt/1 -> Saturation/1
  ObjectVYFilt/1 -> Divide/1
  Fcn/1 -> Object_VYVXAngle0/1

== system PubIfDecisionTOS_MDL/TOS_20201112/TOS_2012080320/TOS/AEB/TOS_AEBLong/AEBLong_Confirm/AEBLong/AEBLong_TrgConfirm/AEBLongTrgJudg/TOS_AEBLong_TargetMovingDir/ObjMovingDirSignalProcessing1/MappingObjInCurveLaneVXVY/ObjectInCurveLaneMappingVXVY/Object_MappingVXVYCalculate/If Action Subsystem1/MappingVX_VY ==
  Object_VX : Inport
  Object_VY : Inport  Port=2
  sinc1 : Inport  Port=3  OutDataTypeStr=single
  cosc1 : Inport  Port=4  OutDataTypeStr=single
  Add : Sum  OutDataTypeStr=single
  Add1 : Sum  Inputs=+-  OutDataTypeStr=single
  Bus Creator : BusCreator  Inputs=4
  Bus Selector : BusSelector  OutputSignals=cosc1,Object_VX
  Bus Selector1 : BusSelector  OutputSignals=sinc1,Object_VY
  Bus Selector2 : BusSelector  OutputSignals=cosc1,Object_VY
  Bus Selector3 : BusSelector  OutputSignals=sinc1,Object_VX
  Product{,1..3} (4 alike) : Product
  MappingVX : Outport
  MappingVY : Outport  Port=2
  wires:
  Object_VX/1 -> Bus Creator/1  "Object_VX"
  Object_VY/1 -> Bus Creator/2  "Object_VY"
  sinc1/1 -> Bus Creator/3  "sinc1"
  cosc1/1 -> Bus Creator/4  "cosc1"
  Bus Selector/1 -> Product/1  "<cosc1>"
  Bus Selector/2 -> Product/2  "<Object_VX>"
  Bus Selector1/1 -> Product1/1  "<sinc1>"
  Bus Selector1/2 -> Product1/2  "<Object_VY>"
  Product/1 -> Add/1
  Product1/1 -> Add/2
  Add/1 -> MappingVX/1
  Bus Selector2/1 -> Product2/1  "<cosc1>"
  Bus Selector2/2 -> Product2/2  "<Object_VY>"
  Bus Creator/1 -> Bus Selector/1, Bus Selector2/1, Bus Selector3/1, Bus Selector1/1
  Bus Selector3/1 -> Product3/1  "<sinc1>"
  Bus Selector3/2 -> Product3/2  "<Object_VX>"
  Product2/1 -> Add1/1
  Product3/1 -> Add1/2
  Add1/1 -> MappingVY/1

== system PubIfDecisionTOS_MDL/TOS_20201112/TOS_2012080320/TOS/AEB/TOS_AEBLong/AEBLong_Confirm/AEBLong/AEBLong_TrgConfirm/AEBLongTrgJudg/TOS_AEBLong_TargetMovingDir/ObjMovingDirSignalProcessing1/MappingObjInCurveLaneVXVY/ObjectInCurveLaneMappingVXVY/Object_MappingVXVYCalculate/If Action Subsystem1/cosC1Calculate_Taylor ==
  note: cosx=1-(x^2)/2
  C1_BaseObjDx : Inport  OutDataTypeStr=single
  Add : Sum  OutDataTypeStr=single
  Constant : Constant  OutDataTypeStr=single
  Gain : Gain  Gain=-0.5  OutDataTypeStr=single
  Math Function : Math  Operator=square  SignedPower=on  OutDataTypeStr=single  SaturateOnIntegerOverflow=on
  cosC1 : Outport  OutDataTypeStr=single
  wires:
  Constant/1 -> Add/2
  C1_BaseObjDx/1 -> Math Function/1
  Math Function/1 -> Gain/1
  Gain/1 -> Add/1
  Add/1 -> cosC1/1

== system PubIfDecisionTOS_MDL/TOS_20201112/TOS_2012080320/TOS/AEB/TOS_AEBLong/AEBLong_Confirm/AEBLong/AEBLong_TrgConfirm/AEBLongTrgJudg/TOS_AEBLong_TargetMovingDir/ObjMovingDirSignalProcessing1/MappingObjInCurveLaneVXVY/ObjectInCurveLaneMappingVXVY/Object_MappingVXVYCalculate/If Action Subsystem1/sinC1Calculate_Taylor ==
  note: sinx=x-(x^3)/6
  C1_BaseObjDx : Inport
  Add : Sum  Inputs=+-  OutDataTypeStr=single
  Constant : Constant  Value=3  OutDataTypeStr=single
  Gain : Gain  Gain=0.167  OutDataTypeStr=single
  Math Function : Math  Operator=pow  SignedPower=on  OutputSignalType=real  SaturateOnIntegerOverflow=on
  sinC1 : Outport  OutDataTypeStr=single
  wires:
  C1_BaseObjDx/1 -> Add/1, Math Function/1
  Constant/1 -> Math Function/2
  Math Function/1 -> Gain/1
  Gain/1 -> Add/2
  Add/1 -> sinC1/1

== matlab function PubIfDecisionTOS_MDL/TOS_20201112/TOS_2012080320/PIL_1029/BoundaryCalculat/ObjectToCenterLine_dyc/LeftLane/PIL_ObjectToCenterLine_dy_Filt/PIL_ObjectToCenterLine_dy/Subsystem/ObjectToCenterLine_dyFilit ==
  data: ObjectID_Filt_K1 input uint8; ObjectToCenterLine_dy_Filt_K1 input single; ObjectToCenterLine_dy input single; ObjectToCenterLine_dy_Filt output single; Object_ID input uint8; TOS_OFMObjValid_Flag input; P_TOS_PIL_ObjectToCenterLine_dy_CutInUpperLimit input single; P_TOS_PIL_ObjectToCenterLine_dy_CutInDeclineLimit input; Iterator_Num input int32
function ObjectToCenterLine_dy_Filt = fcn(ObjectID_Filt_K1,ObjectToCenterLine_dy_Filt_K1,ObjectToCenterLine_dy,...
    Object_ID,TOS_OFMObjValid_Flag,P_TOS_PIL_ObjectToCenterLine_dy_CutInUpperLimit,P_TOS_PIL_ObjectToCenterLine_dy_CutInDeclineLimit, Iterator_Num)

% Iterator_Num = uint8(80);
% K_FiltingParmet_RightLanepil=single(0);
ObjectToCenterLine_dy_Filt = single(0);


if  Object_ID ~=uint8(0) && TOS_OFMObjValid_Flag~=uint8(0)
        for  i=1: int32(Iterator_Num)
            if   ObjectID_Filt_K1(i) == Object_ID && ObjectID_Filt_K1(i)~=uint8(0)  && Object_ID~=uint8(0)   % 目标当前Object_ID 与历史值ObjectID_Filt_K1相同时；滤波处理

                    if ObjectToCenterLine_dy > ObjectToCenterLine_dy_Filt_K1(i) 
                          ObjectToCenterLine_dy_Filt = ObjectToCenterLine_dy_Filt_K1(i) + ...
                          P_TOS_PIL_ObjectToCenterLine_dy_CutInUpperLimit*( ObjectToCenterLine_dy - ObjectToCenterLine_dy_Filt_K1(i)); 
                    else
                         ObjectToCenterLine_dy_Filt = ObjectToCenterLine_dy_Filt_K1(i) + ...
                          P_TOS_PIL_ObjectToCenterLine_dy_CutInDeclineLimit*( ObjectToCenterLine_dy - ObjectToCenterLine_dy_Filt_K1(i)); 
                    end

                    break;
            else
                if i==Iterator_Num    % 如果当前Object_ID首次出现；输出当前值为ObjectToCenterLine_dy_Filt
                    ObjectToCenterLine_dy_Filt = ObjectToCenterLine_dy;        
                else
                    ObjectToCenterLine_dy_Filt = ObjectToCenterLine_dy;  
                end
            end 
        end
else
      ObjectToCenterLine_dy_Filt = ObjectToCenterLine_dy;  
end

== matlab function PubIfDecisionTOS_MDL/TOS_20201112/TOS_2012080320/PIL_1029/BoundaryCalculat/ObjectToCenterLine_dyc/RightLane/PIL_ObjectToCenterLine_dy_Filt/PIL_ObjectToCenterLine_dy/Subsystem/ObjectToCenterLine_dyFilit ==
  data: ObjectID_Filt_K1 input uint8; ObjectToCenterLine_dy_Filt_K1 input single; ObjectToCenterLine_dy input single; ObjectToCenterLine_dy_Filt output single; Object_ID input uint8; TOS_OFMObjValid_Flag input; P_TOS_PIL_ObjectToCenterLine_dy_CutInUpperLimit input single; P_TOS_PIL_ObjectToCenterLine_dy_CutInDeclineLimit input; Iterator_Num input int32
function ObjectToCenterLine_dy_Filt = fcn(ObjectID_Filt_K1,ObjectToCenterLine_dy_Filt_K1,ObjectToCenterLine_dy,...
    Object_ID,TOS_OFMObjValid_Flag,P_TOS_PIL_ObjectToCenterLine_dy_CutInUpperLimit,P_TOS_PIL_ObjectToCenterLine_dy_CutInDeclineLimit, Iterator_Num)

% Iterator_Num = uint8(80);
% K_FiltingParmet_RightLanepil=single(0);
ObjectToCenterLine_dy_Filt = single(0);


if  Object_ID ~=uint8(0) && TOS_OFMObjValid_Flag~=uint8(0)
        for  i=1: int32(Iterator_Num)
            if   ObjectID_Filt_K1(i) == Object_ID && ObjectID_Filt_K1(i)~=uint8(0)  && Object_ID~=uint8(0)   % 目标当前Object_ID 与历史值ObjectID_Filt_K1相同时；滤波处理

                    if ObjectToCenterLine_dy > ObjectToCenterLine_dy_Filt_K1(i) 
                          ObjectToCenterLine_dy_Filt = ObjectToCenterLine_dy_Filt_K1(i) + ...
                          P_TOS_PIL_ObjectToCenterLine_dy_CutInUpperLimit*( ObjectToCenterLine_dy - ObjectToCenterLine_dy_Filt_K1(i)); 
                    else
                         ObjectToCenterLine_dy_Filt = ObjectToCenterLine_dy_Filt_K1(i) + ...
                          P_TOS_PIL_ObjectToCenterLine_dy_CutInDeclineLimit*( ObjectToCenterLine_dy - ObjectToCenterLine_dy_Filt_K1(i)); 
                    end

                    break;
            else
                if i==Iterator_Num    % 如果当前Object_ID首次出现；输出当前值为ObjectToCenterLine_dy_Filt
                    ObjectToCenterLine_dy_Filt = ObjectToCenterLine_dy;        
                else
                    ObjectToCenterLine_dy_Filt = ObjectToCenterLine_dy;  
                end
            end 
        end
else
      ObjectToCenterLine_dy_Filt = ObjectToCenterLine_dy;  
end

== matlab function PubIfDecisionTOS_MDL/TOS_20201112/TOS_2012080320/PIL_1029/BoundaryCalculat/ObjectToCenterLine_dyc/SameLane/PIL_ObjectToCenterLine_dy_Filt/PIL_ObjectToCenterLine_dy/Subsystem/ObjectToCenterLine_dyFilit ==
  data: ObjectID_Filt_K1 input uint8; ObjectToCenterLine_dy_Filt_K1 input single; ObjectToCenterLine_dy input single; ObjectToCenterLine_dy_Filt output single; Object_ID input uint8; TOS_OFMObjValid_Flag input; P_TOS_PIL_ObjectToCenterLine_dy_CutInUpperLimit input single; P_TOS_PIL_ObjectToCenterLine_dy_CutInDeclineLimit input; Iterator_Num input int32
function ObjectToCenterLine_dy_Filt = fcn(ObjectID_Filt_K1,ObjectToCenterLine_dy_Filt_K1,ObjectToCenterLine_dy,...
    Object_ID,TOS_OFMObjValid_Flag,P_TOS_PIL_ObjectToCenterLine_dy_CutInUpperLimit,P_TOS_PIL_ObjectToCenterLine_dy_CutInDeclineLimit, Iterator_Num)

% Iterator_Num = uint8(80);
% K_FiltingParmet_RightLanepil=single(0);
ObjectToCenterLine_dy_Filt = single(0);


if  Object_ID ~=uint8(0) && TOS_OFMObjValid_Flag~=uint8(0)
        for  i=1: int32(Iterator_Num)
            if   ObjectID_Filt_K1(i) == Object_ID && ObjectID_Filt_K1(i)~=uint8(0)  && Object_ID~=uint8(0)   % 目标当前Object_ID 与历史值ObjectID_Filt_K1相同时；滤波处理

                    if ObjectToCenterLine_dy > ObjectToCenterLine_dy_Filt_K1(i) 
                          ObjectToCenterLine_dy_Filt = ObjectToCenterLine_dy_Filt_K1(i) + ...
                          P_TOS_PIL_ObjectToCenterLine_dy_CutInUpperLimit*( ObjectToCenterLine_dy - ObjectToCenterLine_dy_Filt_K1(i)); 
                    else
                         ObjectToCenterLine_dy_Filt = ObjectToCenterLine_dy_Filt_K1(i) + ...
                          P_TOS_PIL_ObjectToCenterLine_dy_CutInDeclineLimit*( ObjectToCenterLine_dy - ObjectToCenterLine_dy_Filt_K1(i)); 
                    end

                    break;
            else
                if i==Iterator_Num    % 如果当前Object_ID首次出现；输出当前值为ObjectToCenterLine_dy_Filt
                    ObjectToCenterLine_dy_Filt = ObjectToCenterLine_dy;        
                else
                    ObjectToCenterLine_dy_Filt = ObjectToCenterLine_dy;  
                end
            end 
        end
else
      ObjectToCenterLine_dy_Filt = ObjectToCenterLine_dy;  
end
